simulink model "Hybrid_P2_Parallel_ETE"  (R2017b)
settings: Solver=FixedStepAuto  StartTime=0.0  StopTime=length(Speed)  FixedStep=0.01  MaxStep=0.01  RelTol=1e-3  EnableMultiTasking=on
PostLoadFcn:
  | , if any(exist('dsrtsu_mdlpostloadfcn', 'file') == [2, 3, 6]), try dsrtsu_mdlpostloadfcn('Execute', bdroot); catch fprintf('Error in PostLoadFcn (dsrtsu_mdlpostloadfcn) for model "%s":\n %s\n', bdroot, lasterr); end, end,
undefined symbols (not defined in the file): Actuators, APP1_OOR, APP2_OOR, APP_Mismatch, Brk_Flt, cal, ClutchEngag, CycLength, CycNmb, DiscIntNeverNeededParam, eng, Engine, EngOverTemp, ENGTRQ_MSMCH_Degraded_CP, ENGTRQ_MSMCH_ErrCritical_CP, ENGTRQ_MSMCH_LimpHome_CP, EngTrqMismatch, ess, ESSOverTemp, gb, Gearbox, KeyPos_Flt, lib_Actuators, lib_EMachine_2017a, lib_Sensors_2017a, Loss, LossCAN, Machine, MCUOverTemp, mot, MotDirMismatch, MotOverTemp, MotTrqMismatch, PRNDL_Flt, Ratio, RegenFault, Scope_new, Scopes1, Sensors, Spd, StopIndex, t_amb, time, tloop
libraries: simulink x117, EC2_libraries x9, powerlib_meascontrol x2, CalculationGallon x1, lib_Chassis x1, lib_DCDC x1, lib_Differential x1, lib_HVESS x1, lib_Engine x1, lib_OBC x1, lib_Transmission x1, Transmission_Validation x1
(part 3 of 10)

== system Hybrid_P2_Parallel_ETE/Camaro Plant Model/Scopes1/AxlTrq_to_EngTrq2/Ratio Filter ==
  Ratio : Inport
  Abs : Abs
  Compare To Zero : simulink/Logic and Bit Operations/Compare To Zero  relop===  OutDataTypeStr=boolean
  Constant : Constant  Value=cal.Time.TrnsOvrllEstTrqRatioSwitch
  Mature_Delay : EC2_libraries/Mature_Delay
      settings: SourceProductName=The database C:\Users\vrajm\AppData\Roaming\MathWorks\MATLAB\R2017b\slblocks_master.db is locked, or a table in the database is locked. (database is locked)
  Memory1 : Memory  InitialCondition=1
  Switch1 : Switch  Threshold=1
  Switch2 : Switch  Threshold=1
  Filtered_Ratio : Outport
  wires:
  Switch2/1 -> Memory1/1, Filtered_Ratio/1  "gear_ratio"
  Memory1/1 -> Switch1/3
  Mature_Delay/1 -> Switch1/2
  Constant/1 -> Mature_Delay/2
  Switch1/1 -> Switch2/1
  Abs/1 -> Switch2/3, Switch1/1
  Compare To Zero/1 -> Switch2/2, Mature_Delay/1
  Ratio/1 -> Abs/1, Compare To Zero/1

== system Hybrid_P2_Parallel_ETE/Camaro Plant Model/Scopes1/AxlTrq_to_MtrTrq2/Ratio Filter ==
  Ratio : Inport
  Abs : Abs
  Compare To Zero : simulink/Logic and Bit Operations/Compare To Zero  relop===  OutDataTypeStr=boolean
  Constant : Constant  Value=cal.Time.TrnsOvrllEstTrqRatioSwitch
  Mature_Delay : EC2_libraries/Mature_Delay
      settings: SourceProductName=The database C:\Users\vrajm\AppData\Roaming\MathWorks\MATLAB\R2017b\slblocks_master.db is locked, or a table in the database is locked. (database is locked)
  Memory1 : Memory  InitialCondition=1
  Switch1 : Switch  Threshold=1
  Switch2 : Switch  Threshold=1
  Filtered_Ratio : Outport
  wires:
  Switch2/1 -> Memory1/1, Filtered_Ratio/1  "gear_ratio"
  Memory1/1 -> Switch1/3
  Mature_Delay/1 -> Switch1/2
  Constant/1 -> Mature_Delay/2
  Switch1/1 -> Switch2/1
  Abs/1 -> Switch2/3, Switch1/1
  Compare To Zero/1 -> Switch2/2, Mature_Delay/1
  Ratio/1 -> Abs/1, Compare To Zero/1

== system Hybrid_P2_Parallel_ETE/Camaro Plant Model/Scopes1/Subsystem/StopCondition  ==
  note: Change the Cycle repeating to triggering repeatition,
      | and add the cycle repeated numbers
  BMS_SOC : Inport
  Gallon_fuel : Inport  Port=2
  10 gallons : simulink/Logic and Bit Operations/Compare To Constant  relop=>=  const=10  OutDataTypeStr=boolean
  Clock : Clock
  Compare To Constant2 : simulink/Logic and Bit Operations/Compare To Constant  relop===  const=4  OutDataTypeStr=boolean
  Constant : Constant  Value=CycNmb
  Constant1 : Constant  Value=0
  Constant2 : Constant  Value=StopIndex
  Constant3 : Constant  Value=CycLength
  Multiport Switch : MultiPortSwitch  Inputs=4
  Product : Product
  Relational Operator : RelationalOperator  Operator===  OutDataTypeStr=boolean  RndMeth=Simplest
  Stop Simulation : Stop
  "stop " : Subsystem
  wires:
  Constant3/1 -> Product/2
  Product/1 -> Relational Operator/2
  Constant1/1 -> Multiport Switch/5
  Relational Operator/1 -> Multiport Switch/4
  Constant/1 -> Product/1
  Gallon_fuel/1 -> 10 gallons/1
  Compare To Constant2/1 -> Multiport Switch/2
  "stop "/1(Out1) -> Compare To Constant2/1
  10 gallons/1 -> Multiport Switch/3
  BMS_SOC/1 -> "stop "/1(In1)
  Constant2/1 -> Multiport Switch/1
  Multiport Switch/1 -> Stop Simulation/1
  Clock/1 -> Relational Operator/1

== system Hybrid_P2_Parallel_ETE/Camaro Plant Model/Transmission/Inputs/Analog_fromHCU ==
  Outputs : Outport
  wires:
  [Analog] -> Outputs/1

== system Hybrid_P2_Parallel_ETE/Camaro Plant Model/Transmission/Inputs/CAN_fromHCU ==
  Outputs : Outport
  wires:
  [HCU_to_VEH_CAN] -> Outputs/1

== system Hybrid_P2_Parallel_ETE/Camaro Plant Model/Transmission/Inputs/Digital_fromHCU ==
  Outputs : Outport
  wires:
  [Digital] -> Outputs/1

== system Hybrid_P2_Parallel_ETE/Camaro Plant Model/Transmission/Soft TCM/6L45 Logic/Gearbox_Control.Shift_Schedule.PlotShiftSchedule ==
  f : TriggerPort  TriggerType=function-call  VariantControl=Variant
      settings: CopyFcn=Stateflow.SLINSF.SimulinkMan.removeBlockPreDeleteFcn  PreDeleteFcn=Stateflow.SLINSF.SimulinkMan.unsafePredeleteFcn
  Subsystem : Subsystem
      settings: OpenFcn=|
      | figure;
      | PlotGearShiftSchedule(Gearbox.L45.PedalPositions,Gearbox.L45.UpShiftSpeeds,Gearbox.L45.DownShiftSpeeds,'6L45')
      mask Display: disp('Plot')

== system Hybrid_P2_Parallel_ETE/Camaro Plant Model/Transmission/Soft TCM/6L45 Logic/Gearbox_Control.Shift_Schedule.calc_down ==
  Gear : Inport
  APP : Inport  Port=2
  f : TriggerPort  TriggerType=function-call  VariantControl=Variant
      settings: CopyFcn=Stateflow.SLINSF.SimulinkMan.removeBlockPreDeleteFcn  PreDeleteFcn=Stateflow.SLINSF.SimulinkMan.unsafePredeleteFcn
  Calculate Downshift Threshold : Lookup2D  RowIndex=gb.ctrl.dmd.init.gear_dnshift.idx1_lin_accel  ColumnIndex=[2,3,4,5,6,7,8]  Table=gb.ctrl.dmd.init.gear_dnshift.map'  LookUpMeth=Interpolation-Use End Values
  down_th : Outport
  wires:
  Calculate Downshift Threshold/1 -> down_th/1
  Gear/1 -> Calculate Downshift Threshold/2
  APP/1 -> Calculate Downshift Threshold/1

== system Hybrid_P2_Parallel_ETE/Camaro Plant Model/Transmission/Soft TCM/6L45 Logic/Gearbox_Control.Shift_Schedule.calc_up ==
  Gear : Inport
  APP : Inport  Port=2
  f : TriggerPort  TriggerType=function-call  VariantControl=Variant
      settings: CopyFcn=Stateflow.SLINSF.SimulinkMan.removeBlockPreDeleteFcn  PreDeleteFcn=Stateflow.SLINSF.SimulinkMan.unsafePredeleteFcn
  Calculate Upshift Threshold : Lookup2D  RowIndex=gb.ctrl.dmd.init.gear_upshift.idx1_lin_accel  ColumnIndex=[1,2,3,4,5,6,7]  Table=gb.ctrl.dmd.init.gear_upshift.map'  LookUpMeth=Interpolation-Use End Values
  up_th : Outport
  wires:
  Calculate Upshift Threshold/1 -> up_th/1
  APP/1 -> Calculate Upshift Threshold/1
  Gear/1 -> Calculate Upshift Threshold/2

== system Hybrid_P2_Parallel_ETE/Camaro Plant Model/Transmission/Soft TCM/6L45 Logic/Torque_Converter_Control.calc_lockup ==
  Gear : Inport
  APP : Inport  Port=2
  f : TriggerPort  TriggerType=function-call  VariantControl=Variant
      settings: CopyFcn=Stateflow.SLINSF.SimulinkMan.removeBlockPreDeleteFcn  PreDeleteFcn=Stateflow.SLINSF.SimulinkMan.unsafePredeleteFcn
  Calculate Lockup Threshold : Lookup2D  RowIndex=cpl.ctrl.init.trqconv_lockup.idx1_lin_accel  ColumnIndex=cpl.ctrl.init.trqconv_lockup.idx2_gear  Table=cpl.ctrl.init.trqconv_lockup.map  LookUpMeth=Interpolation-Use End Values
  lockup_th : Outport
  wires:
  Calculate Lockup Threshold/1 -> lockup_th/1
  APP/1 -> Calculate Lockup Threshold/1
  Gear/1 -> Calculate Lockup Threshold/2

== system Hybrid_P2_Parallel_ETE/Camaro Plant Model/Transmission/Soft TCM/6L45 Logic/Torque_Converter_Control.calc_unlock ==
  Gear : Inport
  APP : Inport  Port=2
  f : TriggerPort  TriggerType=function-call  VariantControl=Variant
      settings: CopyFcn=Stateflow.SLINSF.SimulinkMan.removeBlockPreDeleteFcn  PreDeleteFcn=Stateflow.SLINSF.SimulinkMan.unsafePredeleteFcn
  Calculate Unlock Threshold : Lookup2D  RowIndex=cpl.ctrl.init.trqconv_unlock.idx1_lin_accel  ColumnIndex=cpl.ctrl.init.trqconv_unlock.idx2_gear  Table=cpl.ctrl.init.trqconv_unlock.map  LookUpMeth=Interpolation-Use End Values
  unlock_th : Outport
  wires:
  Calculate Unlock Threshold/1 -> unlock_th/1
  APP/1 -> Calculate Unlock Threshold/1
  Gear/1 -> Calculate Unlock Threshold/2

== system Hybrid_P2_Parallel_ETE/Camaro Plant Model/Transmission/Transmission Plant/ Actuators ==
  In1 : Inport
  Bus Selector : BusSelector  OutputSignals=TransEstGear,LockupCmd
  Out2 : Outport
  Out5 : Outport  Port=2
  wires:
  In1/1 -> Bus Selector/1
  Bus Selector/1 -> Out2/1  "<TransEstGear>"
  Bus Selector/2 -> Out5/1  "<LockupCmd>"

== system Hybrid_P2_Parallel_ETE/Camaro Plant Model/Transmission/Transmission Plant/Gearbox ==
  TransEstGear : Inport
  gb_trq_in gb_inertia_in : Inport  Port=2
  gb_spd_out : Inport  Port=3
  Bus Creator : BusCreator  Inputs=2
  Bus Selector : BusSelector  OutputSignals=tc_trq_out,tc_inertia_out
  Engine Inertia : Constant  Value=Engine.Inertia
  Gear : Lookup  InputValues=gb.plant.init.gear.idx1_shifter  Table=gb.plant.init.gear.idx2_gear  LookUpMeth=Interpolation-Use End Values  OutDataTypeStr=double  SaturateOnIntegerOverflow=on
  Inertia Calculation : Subsystem
  Memory : Memory
  Speed Calculation : Subsystem
  Subsystem : Subsystem
  To Workspace : ToWorkspace  VariableName=TOSS  SampleTime=-1
  Torque calculation : Subsystem
  gear ratio table : Lookup  InputValues=gb.plant.init.ratio.idx1_gear  Table=gb.plant.init.ratio.map  LookUpMeth=Interpolation-Use End Values  SaturateOnIntegerOverflow=on
  "shaftspeed " : lib_Transmission/Transmission/Transmission Plant/Gearbox/shaftspeed 
  gb_trq_out gb_inertia_out : Outport
  gb_spd_in : Outport  Port=2
  tag scope: gb_gear=global, gb_inertia_in=global, gb_inertia_out=global, gb_spd_in=global, gb_spd_out=global, gb_trq_in=global, gb_trq_out=global, gb_trq_ratio=global
  wires:
  Bus Selector/2 -> Inertia Calculation/1(Inertia_in), Speed Calculation/4(Inertia Input)  "<tc_inertia_out>"
  Engine Inertia/1 -> [gb_inertia_in]
  Subsystem/1(Out1) -> [gb_trq_out], Bus Creator/1  "gb_trq_out"
  Torque calculation/1(torque_out) -> Subsystem/1(In1), Subsystem/2(In2)  "gb_trq_out"
  Memory/1 -> Gear/1
  gear ratio table/1 -> [gb_trq_ratio]
  Bus Creator/1 -> gb_trq_out gb_inertia_out/1
  Inertia Calculation/1(Inertia) -> Bus Creator/2, [gb_inertia_out]  "gb_inertia_out"
  gb_trq_in gb_inertia_in/1 -> Bus Selector/1
  Gear/1 -> Torque calculation/2(gear number), Inertia Calculation/2(gear number), gear ratio table/1, [gb_gear], Speed Calculation/1(gear number)
  Bus Selector/1 -> Torque calculation/3(" input torque"), Speed Calculation/3(torque input), [gb_trq_in]  "<tc_trq_out>"
  TransEstGear/1 -> Memory/1
  Speed Calculation/1(Speed) -> gb_spd_in/1, "shaftspeed "/1, [gb_spd_in]
  gb_spd_out/1 -> Speed Calculation/2(spd out), "shaftspeed "/2, [gb_spd_out], To Workspace/1, Torque calculation/1(speed out)

== system Hybrid_P2_Parallel_ETE/Camaro Plant Model/Transmission/Transmission Plant/Sensors ==
  In2 : Inport
  In3 : Inport  Port=2
  In4 : Inport  Port=3
  In5 : Inport  Port=4
  In6 : Inport  Port=5
  In7 : Inport  Port=6
  In1 : Inport  Port=7
  Bus Creator : BusCreator  Inputs=7
  Out1 : Outport
  wires:
  In1/1 -> Bus Creator/7  "gb_trq_ratio"
  Bus Creator/1 -> Out1/1
  In2/1 -> Bus Creator/1  "impeller_spd_rads"
  In4/1 -> Bus Creator/3  "tc_trq_in"
  In5/1 -> Bus Creator/4  "tc_trq_out"
  In3/1 -> Bus Creator/2  "turbine_spd_rads"
  In6/1 -> Bus Creator/5  "TrnsOutShftAngVel"
  In7/1 -> Bus Creator/6  "TrnsOutShftTrq"

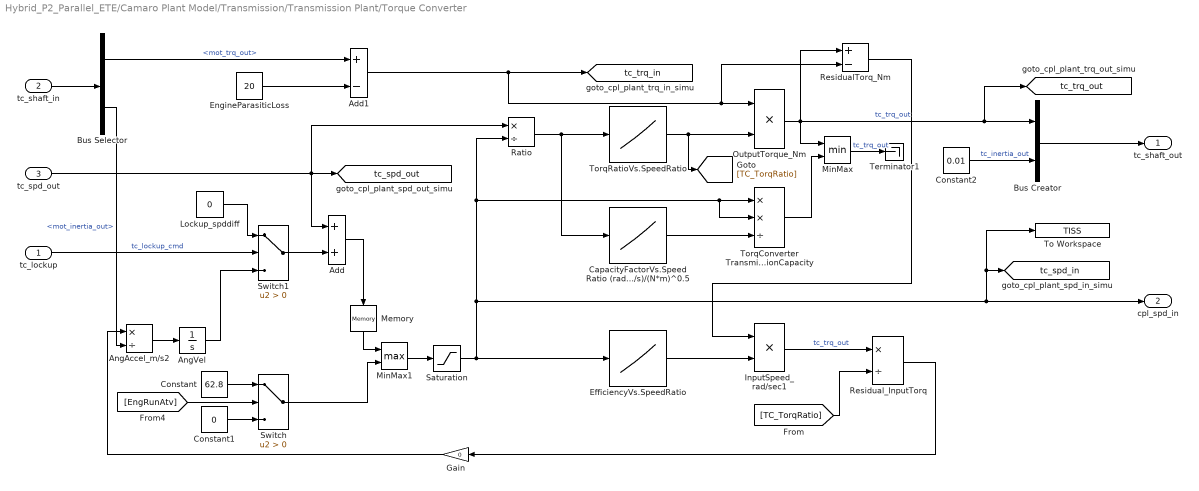
== system Hybrid_P2_Parallel_ETE/Camaro Plant Model/Transmission/Transmission Plant/Torque Converter ==
  tc_lockup : Inport
  tc_shaft_in : Inport  Port=2
  tc_spd_out : Inport  Port=3
  Add : Sum
  Add1 : Sum  Inputs=+-
  AngAccel_m/s2 : Product  Inputs=*/
  AngVel : Integrator
  Bus Creator : BusCreator  Inputs=2
  Bus Selector : BusSelector  OutputSignals=mot_trq_out,mot_inertia_out
  CapacityFactorVs.SpeedRatio (rad/s)/(N*m)^0.5 : Lookup_n-D  NumberOfTableDimensions=1  BreakpointsForDimension1=[0 0.50 0.60 0.70 0.80 0.87 0.92 0.94 0.96 0.97]  Table=[12.2938 12.8588 13.1452 13.6285 14.6163 16.2675 19.3503 22.1046 29.9986 50.00]  InternalRulePriority=Speed  RndMeth=Simplest  InputSameDT=on
  Constant : Constant  Value=62.8
  Constant1 : Constant  Value=0
  Constant2 : Constant  Value=0.01
  EfficiencyVs.SpeedRatio : Lookup_n-D  NumberOfTableDimensions=1  BreakpointsForDimension1=[0 0.25 0.50 0.60 0.70 0.80 0.87 0.92 0.94 0.96 0.97 1.0]  Table="[0.10 0.50 0.70 0.8 0.8 0.80  0.85 0.87 0.91 0.95 0.96 0.96]"  InternalRulePriority=Speed  RndMeth=Simplest  InputSameDT=on
  EngineParasiticLoss : Constant  Value=20
  Gain : Gain  Gain=0
  InputSpeed_rad/sec1 : Product  Inputs=**
  Lockup_spddiff : Constant  Value=0
  Memory : Memory  InitialCondition=1
  MinMax : MinMax  Inputs=2
  MinMax1 : MinMax  Function=max  Inputs=2
  OutputTorque_Nm : Product  Inputs=**
  Ratio : Product  Inputs=*/
  ResidualTorq_Nm : Sum  Inputs=+-
  Residual_InputTorq : Product  Inputs=*/
  Saturation : Saturate  UpperLimit=1100  LowerLimit=1
  Switch : Switch  Criteria=u2 > Threshold
  Switch1 : Switch  Criteria=u2 > Threshold
  Terminator1 : Terminator
  To Workspace : ToWorkspace  VariableName=TISS  SampleTime=-1
  TorqConverter TransmissionCapacity : Product  Inputs=**/
  TorqRatioVs.SpeedRatio : Lookup_n-D  NumberOfTableDimensions=1  BreakpointsForDimension1=[0 0.50 0.60 0.70 0.80 0.87 0.92 0.94 0.96 0.97]  Table=[2.2320 1.5462 1.4058 1.2746 1.1528 1.0732 1.0192 0.9983 0.9983 0.9983]  InternalRulePriority=Speed  RndMeth=Simplest  InputSameDT=on
  tc_shaft_out : Outport
  cpl_spd_in : Outport  Port=2
  tag scope: tc_spd_in=global, tc_spd_out=global, tc_trq_in=global, tc_trq_out=global
  wires:
  Lockup_spddiff/1 -> Switch1/1
  Switch1/1 -> Add/2
  Bus Selector/1 -> Add1/1  "<mot_trq_out>"
  Constant1/1 -> Switch/3
  Constant/1 -> Switch/1
  [EngRunAtv] -> Switch/2
  Switch/1 -> MinMax1/2
  MinMax1/1 -> Saturation/1
  Gain/1 -> AngAccel_m/s2/1
  Add/1 -> Memory/1
  tc_spd_out/1 -> Add/1, [tc_spd_out], Ratio/1
  MinMax/1 -> Terminator1/1  "tc_trq_out"
  OutputTorque_Nm/1 -> MinMax/1, [tc_trq_out], Bus Creator/1, ResidualTorq_Nm/1  "tc_trq_out"
  Residual_InputTorq/1 -> Gain/1
  EngineParasiticLoss/1 -> Add1/2
  Memory/1 -> MinMax1/1
  AngVel/1 -> Switch1/3
  AngAccel_m/s2/1 -> AngVel/1
  InputSpeed_rad/sec1/1 -> Residual_InputTorq/1  "tc_trq_out"
  ResidualTorq_Nm/1 -> InputSpeed_rad/sec1/1
  [TC_TorqRatio] -> Residual_InputTorq/2
  TorqConverter TransmissionCapacity/1 -> MinMax/2
  EfficiencyVs.SpeedRatio/1 -> InputSpeed_rad/sec1/2
  Saturation/1 -> EfficiencyVs.SpeedRatio/1, cpl_spd_in/1, To Workspace/1, [tc_spd_in], TorqConverter TransmissionCapacity/1, TorqConverter TransmissionCapacity/2, Ratio/2
  Ratio/1 -> TorqRatioVs.SpeedRatio/1, CapacityFactorVs.SpeedRatio (rad/s)/(N*m)^0.5/1
  CapacityFactorVs.SpeedRatio (rad/s)/(N*m)^0.5/1 -> TorqConverter TransmissionCapacity/3
  TorqRatioVs.SpeedRatio/1 -> [TC_TorqRatio], OutputTorque_Nm/2
  tc_lockup/1 -> Switch1/2  "tc_lockup_cmd"
  Bus Selector/2 -> AngAccel_m/s2/2  "<mot_inertia_out>"
  Bus Creator/1 -> tc_shaft_out/1
  tc_shaft_in/1 -> Bus Selector/1
  Constant2/1 -> Bus Creator/2  "tc_inertia_out"
  Add1/1 -> OutputTorque_Nm/1, ResidualTorq_Nm/2, [tc_trq_in]

== system Hybrid_P2_Parallel_ETE/Controller_with_Transmission_Manager1/HSC/Camaro Fault Detection/Component Diagnostic ==
  note: Component Diagnostics
  note: Component Status Setting Rule
      | xxx_CompStatus could be 0, 1, 2 or 3
      | 0: component needs to be offline
      | 1: component needs torque plant to deliver creep torque
      | 2: component needs torque plant to limit maximum torque delivery
      | 3: component needs torque plant to operate normally
  SignalDiag : Inport
  Bus Creator : BusCreator  Inputs=6
  Driver Input Diagnostic : Subsystem
  ESS Component Diagnostic : Subsystem
  Engine Component Diagnostic : Subsystem
  Override Driver Status : Subsystem
  Override ESS Status : Subsystem
  Override Engine Status : Subsystem
  Override TCM Status : Subsystem
  Transmission Component Diagnostic : Subsystem
  CompDiag : Outport
  wires:
  Engine Component Diagnostic/2(Out2) -> Bus Creator/4  "EngTrqMismchType"
  Override Driver Status/1(Out1) -> Bus Creator/1  "Driver_Input_Status"
  Override TCM Status/1(Out1) -> Bus Creator/5  "TCM_Status"
  Override Engine Status/1(Out1) -> Bus Creator/3  "ECM_Status"
  Override ESS Status/1(Out1) -> Bus Creator/2  "BMS_Status"
  Transmission Component Diagnostic/1(Out1) -> Override TCM Status/1(In1)  "TCM_CompDiag"
  Engine Component Diagnostic/1(Out1) -> Override Engine Status/1(In1)  "ECM_CompDiag"
  ESS Component Diagnostic/1(Out1) -> Override ESS Status/1(In1)  "ESS_CompDiag"
  Driver Input Diagnostic/1(Out1) -> Override Driver Status/1(In1)  "Diver_CompDiag"
  Bus Creator/1 -> CompDiag/1
  SignalDiag/1 -> Driver Input Diagnostic/1(In1), ESS Component Diagnostic/1(In1), Bus Creator/6, Transmission Component Diagnostic/1(In1), Engine Component Diagnostic/1(In1)  "RawSig"

== system Hybrid_P2_Parallel_ETE/Controller_with_Transmission_Manager1/HSC/Camaro Fault Detection/Input Conversions ==
  note: These subsystems convert variable types to match those used in the
      | supervisor. In addition, override switches installed on each signal can
      | be used to manually override and signal for testing purposes
  note: Input Conversions and Override Switches
  RawSig : Inport
  BMS_Conversions : Subsystem
  Bus Creator : BusCreator  Inputs=5
  DriverInput_Conversions : Subsystem
  ECM_Conversions : Subsystem
  TCM_Conversions : Subsystem
  VehSig : Outport
  wires:
  TCM_Conversions/1(Out1) -> Bus Creator/4
  ECM_Conversions/1(Out1) -> Bus Creator/3
  RawSig/1 -> BMS_Conversions/1(In1), ECM_Conversions/1(In1), TCM_Conversions/1(In1), Bus Creator/5, DriverInput_Conversions/1(In1)  "RawSig"
  BMS_Conversions/1(Out1) -> Bus Creator/2
  Bus Creator/1 -> VehSig/1  "InputConvAndOvrd"
  DriverInput_Conversions/1(Out1) -> Bus Creator/1

== system Hybrid_P2_Parallel_ETE/Controller_with_Transmission_Manager1/HSC/Camaro Fault Detection/Signal Diagnostic ==
  note: Signal Diagnostics
  note: These subsystems evaluate each signal for proper value range and other checks
  VehSig : Inport
  Bus Creator : BusCreator  Inputs=5
  Driver Signal Diagnostic : Subsystem
  ESS Signal Diagnostic : Subsystem
  Engine Signal Diagnostic : Subsystem
  Subsystem1 : Subsystem
      mask Display: fprintf('Signal Naming Rule')
  Transmission Signal Diagnostic : Subsystem
  SignalDiag : Outport
  wires:
  Bus Creator/1 -> SignalDiag/1  "SignalDiag"
  Transmission Signal Diagnostic/1(Out2) -> Bus Creator/4  "Transmission_SigDiag"
  Engine Signal Diagnostic/1(Engine_SigDiag) -> Bus Creator/3  "Engine_SigDiag"
  ESS Signal Diagnostic/1(ESS_SigDiag) -> Bus Creator/2  "ESS_SigDiag"
  Driver Signal Diagnostic/1(Driver_SigDiag) -> Bus Creator/1  "Driver_SigDiag"
  VehSig/1 -> Transmission Signal Diagnostic/1(Sensors1), Bus Creator/5, Engine Signal Diagnostic/1(Sensors1), Driver Signal Diagnostic/1(Sensors1), ESS Signal Diagnostic/1(Sensors1)

== system Hybrid_P2_Parallel_ETE/Controller_with_Transmission_Manager1/HSC/Driver_Requests/APP_BPP to DrvIntndAxlTrq2 ==
  note: Note:Driver requested Axle Torque Calculation
  note: $Author: fy6949 $
      | $Rev: 577 $
      | $Date: 2017-1-19 08:53:15 -0500  $
  Sensors : Inport
  Diag : Inport  Port=2
  Controls : Inport  Port=3
  Bus Selector : BusSelector  OutputSignals=from_Analog.Driver_APP1,from_CAN.fromVEH_CAN.from_BCM.BrkPdlPos,from_CAN.fromEBCAN.from_ECM.VehSpdAvgDrvn,from_CAN.fromVEH_CAN.from_TCM.TrnGrRat,from_CAN.fromHV_CAN.from_MCU.INV_VCU_01.INV_Speed
  Bus Selector1 : BusSelector  OutputSignals=CompSig.RawSig.Driver_SigDiag.Drv_APP_Agree
  Bus Selector2 : BusSelector  OutputSignals=mode
  Post Driver Intnded Axle Torque : Subsystem
  Terminator : Terminator
  Terminator1 : Terminator
  IntndAxlTrq : Outport
  wires:
  Sensors/1 -> Bus Selector/1
  Controls/1 -> Bus Selector2/1
  Post Driver Intnded Axle Torque/1(IntndAxlTrq) -> IntndAxlTrq/1
  Bus Selector/2 -> Post Driver Intnded Axle Torque/2(BPP)  "<BrkPdlPos>"
  Bus Selector/3 -> Post Driver Intnded Axle Torque/3(VehicleSpeed)  "<VehSpdAvgDrvn>"
  Bus Selector/5 -> Post Driver Intnded Axle Torque/6(Motor_Speed)  "<INV_Speed>"
  Bus Selector/4 -> Post Driver Intnded Axle Torque/4(TransGearRatio)  "<TrnGrRat>"
  Bus Selector/1 -> Post Driver Intnded Axle Torque/1(APP)  "<Driver_APP1>"
  Post Driver Intnded Axle Torque/2(BrkIntndAxlTrq) -> Terminator/1
  Diag/1 -> Bus Selector1/1
  Bus Selector1/1 -> Terminator1/1  "<Drv_APP_Agree>"
  Bus Selector2/1 -> Post Driver Intnded Axle Torque/5(Mode)  "<mode>"

== system Hybrid_P2_Parallel_ETE/Controller_with_Transmission_Manager1/HSC/Powertrain Manager/HV Manager1 ==
  Sensors : Inport
  Controls : Inport  Port=2
  Axiomatic_Output_Manager : Subsystem
  BMS_Manager : Subsystem
  Bus Creator1 : BusCreator  Inputs=4
  DCDC Manager : Subsystem
  Inverter Manager : Subsystem
  OBC_Manager : Subsystem
  BMS_CAN : Outport
  HV_BUS_Status : Outport  Port=2
  OBC_CAN : Outport  Port=3
  OBC_Digital : Outport  Port=4
  BMS_Digital : Outport  Port=5
  Axiomatic_CAN : Outport  Port=6
  tag scope: MCU_CAN=global
  wires:
  Bus Creator1/1 -> [MCU_CAN]
  Inverter Manager/2(MCU_CAN) -> Bus Creator1/2  "MCU_CAN"
  Inverter Manager/1(MCU_Status) -> [MCU_Status], Bus Creator1/1  "MCU_Status"
  Sensors/1 -> BMS_Manager/1(Sensors), DCDC Manager/1(BMSInput), Axiomatic_Output_Manager/1(Sensors), OBC_Manager/2(Sensors), Inverter Manager/2(Sensors)
  [HV_BUS_Status] -> Inverter Manager/1(HV_Bus_Status)  "HV_BUS_Status"
  [HV_BUS_Status] -> Axiomatic_Output_Manager/2(HV_Bus_Status)
  BMS_Manager/2(HV_BUS_Status) -> [HV_BUS_Status], HV_BUS_Status/1  "HV_BUS_Status"
  [HV_BUS_Status] -> OBC_Manager/1(HV_Status)
  OBC_Manager/1(OBC CAN) -> OBC_CAN/1
  OBC_Manager/2(OBC_Digital) -> OBC_Digital/1
  Controls/1 -> BMS_Manager/2(Controls), DCDC Manager/2(In1), DCDC Manager/3(In2), Inverter Manager/3(Control)
  BMS_Manager/1(BMS CAN) -> BMS_CAN/1
  BMS_Manager/3(BMS Digital) -> BMS_Digital/1
  Axiomatic_Output_Manager/1(Axiomatic_CAN) -> Axiomatic_CAN/1
  Inverter Manager/3(MCU_Relay) -> Bus Creator1/3  "MCU_Relay"
  DCDC Manager/1(Out1) -> Bus Creator1/4
  [MCU_Status] -> BMS_Manager/3(In1)

== system Hybrid_P2_Parallel_ETE/Controller_with_Transmission_Manager1/HSC/Powertrain Manager/Output Conversion ==
  In1 : Inport
  In2 : Inport  Port=2
  In3 : Inport  Port=3
  In4 : Inport  Port=4
  In5 : Inport  Port=5
  In8 : Inport  Port=6
  In9 : Inport  Port=7
  In10 : Inport  Port=8
  In11 : Inport  Port=9
  Bus Creator : BusCreator  Inputs=14
  Bus Creator1 : BusCreator  Inputs=9
  Bus Selector2 : BusSelector  OutputSignals=powerMode,EnablePrplsn,ClutchEngage,EngAppReq,EngOnReq,MtrTrqCmdOut,EnableInverter,EngTrqCmd,HV_req,SysPwrMd_0_3,TrnsShftLvrPos,VehSpdAvgDrvn_kph,AccPos_Perc,SportsModeEnable
  Data Type Conversion{,2..3,5..13} (12 alike) : DataTypeConversion
  Memory : Memory
  Out1 : Outport
  wires:
  In10/1 -> Bus Creator1/8
  In9/1 -> Bus Creator1/7
  In8/1 -> Bus Creator1/6
  Memory/1 -> Data Type Conversion/1
  Data Type Conversion13/1 -> Bus Creator/13  "AccPos_Perc"
  Bus Selector2/13 -> Data Type Conversion13/1  "<AccPos_Perc>"
  Data Type Conversion12/1 -> Bus Creator/12  "VehSpdAvgDrvn_kph"
  Bus Selector2/12 -> Data Type Conversion12/1  "<VehSpdAvgDrvn_kph>"
  Data Type Conversion11/1 -> Bus Creator/11  "ShftLvrPos"
  Bus Selector2/11 -> Data Type Conversion11/1  "<TrnsShftLvrPos>"
  In5/1 -> Bus Creator1/5
  Bus Creator/1 -> Bus Creator1/4  "Controls"
  In3/1 -> Bus Creator1/3
  In2/1 -> Bus Creator1/2
  In1/1 -> Bus Creator1/1
  Bus Creator1/1 -> Out1/1
  Data Type Conversion5/1 -> Bus Creator/5  "EngOnReq"
  Data Type Conversion/1 -> Bus Creator/1  "powerMode"
  Data Type Conversion10/1 -> Bus Creator/10  "SysPwrMd"
  Data Type Conversion9/1 -> Bus Creator/9  "HV_req"
  Data Type Conversion8/1 -> Bus Creator/8  "EngTrqCmd"
  Data Type Conversion7/1 -> Bus Creator/7  "Inverter_Enable"
  Data Type Conversion6/1 -> Bus Creator/6  "Torque_Command"
  Bus Selector2/4 -> Bus Creator/4  "<EngAppReq>"
  Data Type Conversion3/1 -> Bus Creator/3  "ClutchEngage"
  Data Type Conversion2/1 -> Bus Creator/2  "EnablePrplsn"
  Bus Selector2/10 -> Data Type Conversion10/1  "<SysPwrMd_0_3>"
  Bus Selector2/9 -> Data Type Conversion9/1  "<HV_req>"
  Bus Selector2/8 -> Data Type Conversion8/1  "<EngTrqCmd>"
  Bus Selector2/7 -> Data Type Conversion7/1  "<EnableInverter>"
  Bus Selector2/6 -> Data Type Conversion6/1  "<MtrTrqCmdOut>"
  Bus Selector2/5 -> Data Type Conversion5/1  "<EngOnReq>"
  Bus Selector2/3 -> Data Type Conversion3/1  "<ClutchEngage>"
  Bus Selector2/2 -> Data Type Conversion2/1  "<EnablePrplsn>"
  Bus Selector2/1 -> Memory/1  "<powerMode>"
  In4/1 -> Bus Selector2/1
  In11/1 -> Bus Creator1/9
  Bus Selector2/14 -> Bus Creator/14  "<SportsModeEnable>"

== system Hybrid_P2_Parallel_ETE/Controller_with_Transmission_Manager1/HSC/Powertrain Manager/Thermal Manager ==
  In2 : Inport
  Bus Creator : BusCreator  Inputs=3
  Bus Creator1 : BusCreator  Inputs=4
  Bus Creator2 : BusCreator  Inputs=4
  Bus Creator3 : BusCreator  Inputs=3
  Bus Creator4 : BusCreator  Inputs=1
  Bus Selector : BusSelector  OutputSignals=from_CAN.fromEBCAN.from_ECM.EngCltTmp,from_CAN.fromHV_CAN.from_BMSHybrid.BMS_Temperatur,from_CAN.fromHV_CAN.from_MCU.INV_VCU_04.INV_InverterTemperature,from_CAN.fromHV_CAN.from_MCU.INV_VCU_04.INV_ElectricMachineTemperature,from_CAN.fromEBCAN.from_ECM.EngRunAtv,from_CAN.fromHV_CAN.from_BMSHybrid.BMS_HYB_02.BMS_IstModus,from_CAN.fromVEH_CAN.from_BCM.SysPwrMd,from_CAN.fromEBCAN.from_ECM.VehSpdAvgDrvn
  Bus Selector3 : BusSelector  OutputSignals=from_CAN.fromHV_CAN.from_BMSHybrid.BMS_HYB_02.BMS_Fehler_Pilot
  Compare To Constant1 : simulink/Logic and Bit Operations/Compare To Constant  relop=>  const=0  OutDataTypeStr=boolean
  Cooling Fan Manger : Subsystem
  Data Type Conversion : DataTypeConversion  OutDataTypeStr=double
  ESS Pump Manger : Subsystem
  MotInv Pump Manger : Subsystem
  Out1 : Outport
  wires:
  Bus Selector/8 -> Bus Creator/3  "<VehSpdAvgDrvn>"
  Bus Selector/7 -> Bus Creator3/3  "<SysPwrMd>"
  Bus Selector/6 -> Bus Creator3/2  "<BMS_IstModus>"
  Bus Selector/5 -> Bus Creator3/1  "<EngRunAtv>"
  Bus Selector/4 -> Bus Creator2/4  "<INV_ElectricMachineTemperature>"
  Bus Selector/3 -> Bus Creator2/3  "<INV_InverterTemperature>"
  Bus Selector/2 -> Bus Creator2/2  "<BMS_Temperatur>"
  Bus Selector/1 -> Bus Creator2/1  "<EngCltTmp>"
  Bus Creator1/1 -> Out1/1  "Thermal_Control"
  Cooling Fan Manger/1(Fan_control) -> Bus Creator1/1  "Fan_Control"
  Bus Creator/1 -> Cooling Fan Manger/1(Temp), ESS Pump Manger/1(ESS_temp), MotInv Pump Manger/1(MotInv_temp)
  ESS Pump Manger/1(ESS_Thermal_Control) -> Bus Creator1/2  "ESS_Pump_Control"
  MotInv Pump Manger/1(MotInvpump_control) -> Bus Creator1/3  "MotMCU_Pump_Control"
  Bus Creator2/1 -> Bus Creator/1  "Temp_Signals"
  Bus Creator3/1 -> Bus Creator/2  "Component_State"
  In2/1 -> Bus Selector3/1, Bus Selector/1
  Bus Selector3/1 -> Compare To Constant1/1  "<BMS_Fehler_Pilot>"
  Bus Creator4/1 -> Bus Creator1/4  "Pump_Commands"
  Data Type Conversion/1 -> Bus Creator4/1  "FuelPump_Disable"
  Compare To Constant1/1 -> Data Type Conversion/1

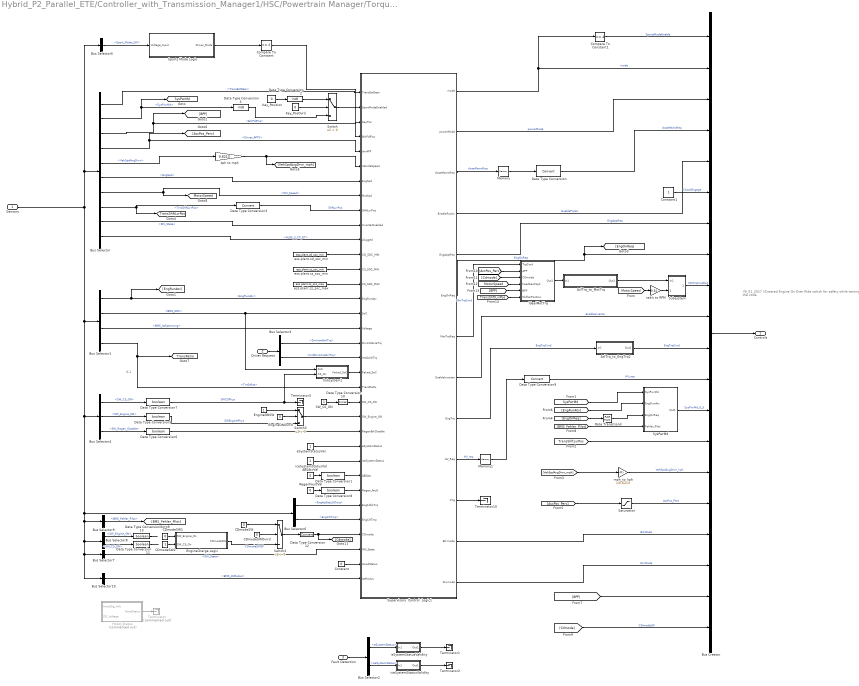
== system Hybrid_P2_Parallel_ETE/Controller_with_Transmission_Manager1/HSC/Powertrain Manager/Torque Distribution1 ==
  note: 0-1
  note: //9_01_2017
      | //Created Engine On Over Ride switch for safety while testing the code
  Sensors : Inport
  Driver Request : Inport  Port=2
  Fault Detection : Inport  Port=3
  ABSAtvVal : Constant  Value=0
  AxlTrq_to_EngTrq2 : Subsystem
  AxlTrq_to_MotTrq : Subsystem
  Bus Creator : BusCreator  Inputs=20
  Bus Selector : BusSelector  OutputSignals=from_CAN.fromVEH_CAN.from_TCM.TransEstGear,from_CAN.fromVEH_CAN.from_BCM.SysPwrMd,from_CAN.fromVEH_CAN.from_BCM.BrkPdlPos,from_Analog.Driver_APP1,from_CAN.fromEBCAN.from_ECM.VehSpdAvgDrvn,from_CAN.fromEBCAN.from_ECM.EngSpd,from_CAN.fromHV_CAN.from_MCU.INV_VCU_01.INV_Speed,from_CAN.fromVEH_CAN.from_TCM.TrnsShftLvrPos,from_CAN.fromHV_CAN.from_MCU.INV_VCU_01.INV_State,from_CAN.fromHV_CAN.from_OBC.NLG5_ST.NLG5_S_CP_DT
  Bus Selector1 : BusSelector  OutputSignals=from_CAN.fromEBCAN.from_ECM.EngRunAtv,from_CAN.fromHV_CAN.from_BMSHybrid.BMS_SOC,from_CAN.fromHV_CAN.from_BMSHybrid.BMS_HYB_02.BMS_IstSpannung,from_CAN.fromVEH_CAN.from_TCM.TrnGrRat
  Bus Selector10 : BusSelector  OutputSignals=from_CAN.fromHV_CAN.from_BMSHybrid.BMS_HYB_02.BMS_IstModus
  Bus Selector2 : BusSelector  OutputSignals=eSystemDiagOut.eSystemStatus,iceSystemDiagOut.iceSystemStatus
  Bus Selector3 : BusSelector  OutputSignals=DrvIntndAxlTrq,FullDrvIntndAxlTrq
  Bus Selector4 : BusSelector  OutputSignals=from_Digital.SW_CS_ON,from_Digital.SW_Engine_ON,from_Digital.SW_Regen_Disable
  Bus Selector5 : BusSelector  OutputSignals=from_Analog.Sport_Mode_SW
  Bus Selector6 : BusSelector  OutputSignals=from_CAN.fromEBCAN.from_ECM.EngActStdyStTorq,from_CAN.fromEBCAN.from_ECM.EngCltTmp
  Bus Selector7 : BusSelector  OutputSignals=from_CAN.fromHV_CAN.from_MCU.INV_VCU_01.INV_State
  Bus Selector8 : BusSelector  OutputSignals=from_Digital.SW_Engine_ON,from_Digital.SW_CS_ON
  Bus Selector9 : BusSelector  OutputSignals=from_CAN.fromHV_CAN.from_BMSHybrid.BMS_HYB_02.BMS_Fehler_Pilot
  CDmodeSW : Constant  Value=0
  CDmodeSW1 : Constant  Value=0
  CDmodeSW2 : Constant
  CDmodeSWOvrrd : Constant  Value=0
  Compare To Constant : simulink/Logic and Bit Operations/Compare To Constant  relop===  const=2  OutDataTypeStr=boolean
  Compare To Constant1 : simulink/Logic and Bit Operations/Compare To Constant  relop===  const=4  OutDataTypeStr=boolean
  Constant : Constant  Value=0
  Constant1 : Constant
  Data Type Conversion{,3,9,12} (4 alike) : DataTypeConversion
  Data Type Conversion{1,5..8,10..11,13} (8 alike) : DataTypeConversion  OutDataTypeStr=boolean
  Data Type Conversion2 : DataTypeConversion  OutDataTypeStr=int8
  Data Type Conversion4 : DataTypeConversion  OutDataTypeStr=int8
  EngineCharge Logic : Stateflow chart  TreatAsAtomicUnit=on
  EngineONOvrrd : Constant  Value=0
  EngineONSW : Constant
  Hood_Status : Subsystem  Commented=on
  IdealMotTrq : Subsystem
  Key_PosOvrd : Constant  Value=0
  Key_Position : Constant  Value=0
  Memory : Memory
  Memory1 : Memory
  Rate Transition3 : RateTransition
  RegenFaultVal : Constant  Value=0
  SW_CS_ON : Constant
  Saturation : Saturate  UpperLimit=100  LowerLimit=0
  Sports Mode Logic : Stateflow chart  TreatAsAtomicUnit=on
  Subsystem : Subsystem
  Subsystem1 : Subsystem
  Supervisory  Control  Logic1 : Stateflow chart  TreatAsAtomicUnit=on
  Switch : Switch  Criteria=u2 > Threshold
  Switch2 : Switch  Criteria=u2 > Threshold
  Switch3 : Switch  Criteria=u2 > Threshold
  SysPwrMd : Subsystem
  Terminator : Terminator  Commented=on
  Terminator{1..3,10} (4 alike) : Terminator
  eSystemStatusVal : Constant
  eSystemStatusValidity : Subsystem
  ess.plant.cd_soc_min : Constant  Value=ess.plant.cd_soc_min
  ess.plant.cs_soc_max : Constant  Value=ess.plant.cs_soc_max
  ess.plant.cs_soc_min : Constant  Value=ess.plant.cs_soc_min
  iceSystemStatusVal : Constant
  iceSystemStatusValidity : Subsystem
  kph to mph : Gain  Gain=0.6213
  mph_to_kph : Gain  Gain=1/0.6213
  rad/s to RPM : Gain  Gain=9.54
  Controls : Outport
  tag scope: MotorSpeed=global, SysPwrMd=global, TransRatio=global, TransShftLvrPos=global
  wires:
  Bus Selector/1 -> Supervisory  Control  Logic1/1(TransEstGear)  "<TransEstGear>"
  Bus Selector/2 -> [SysPwrMd], Data Type Conversion4/1  "<SysPwrMd>"
  Bus Selector/3 -> [BPP], Supervisory  Control  Logic1/4(BrkPdlPos)  "<BrkPdlPos>"
  Bus Selector/4 -> [AccPos_Perc], Supervisory  Control  Logic1/5(drvAPP)  "<Driver_APP1>"
  Bus Selector/5 -> kph to mph/1  "<VehSpdAvgDrvn>"
  Bus Selector/6 -> Supervisory  Control  Logic1/7(EngSpd)  "<EngSpd>"
  Bus Selector/7 -> [MotorSpeed], Supervisory  Control  Logic1/8(MotSpd)  "<INV_Speed>"
  Bus Selector/9 -> Supervisory  Control  Logic1/10(InverterEnabled)  "<INV_State>"
  Bus Selector1/1 -> Supervisory  Control  Logic1/15(EngRunAtv), [EngRunAtv]  "<EngRunAtv>"
  Bus Selector1/2 -> Subsystem1/1(SoC), Supervisory  Control  Logic1/16(SoC)  "<BMS_SOC>"
  ess.plant.cd_soc_min/1 -> Supervisory  Control  Logic1/12(CD_SOC_MIN)
  ess.plant.cs_soc_min/1 -> Supervisory  Control  Logic1/13(CS_SOC_MIN)
  ess.plant.cs_soc_max/1 -> Supervisory  Control  Logic1/14(CS_SOC_MAX)
  Supervisory  Control  Logic1/6(EngOnReq) -> [EngOnReq], Bus Creator/8  "EngOnReq"
  Supervisory  Control  Logic1/8(EnableInverter) -> Bus Creator/10  "EnableInverter"
  Supervisory  Control  Logic1/4(EnablePrplsn) -> Bus Creator/5  "EnablePrplsn"
  Supervisory  Control  Logic1/3(closeMaincReq) -> Memory/1  "closeMaincReq"
  Supervisory  Control  Logic1/2(powerMode) -> Bus Creator/3  "powerMode"
  Supervisory  Control  Logic1/1(mode) -> Compare To Constant1/1, Bus Creator/2  "mode"
  [EngOnReq] -> Rate Transition3/1
  [EngRunAtv] -> SysPwrMd/2(EngRunAtv)
  [SysPwrMd] -> SysPwrMd/1(SysPwrMd)
  Compare To Constant/1 -> Supervisory  Control  Logic1/2(SportModeEnabled)
  Data Type Conversion3/1 -> Supervisory  Control  Logic1/9(ShftLvrPos)  "ShftLvrPos"
  Bus Selector/8 -> [TransShftLvrPos], Data Type Conversion3/1  "<TrnsShftLvrPos>"
  kph to mph/1 -> [VehSpdAvgDrvn_mph], Supervisory  Control  Logic1/6(VehicleSpeed)
  Bus Creator/1 -> Controls/1
  Supervisory  Control  Logic1/9(EngTrq) -> AxlTrq_to_EngTrq2/1(In1)  "EngTrqCmd"
  Bus Selector1/4 -> Supervisory  Control  Logic1/21(TransRatio), [TransRatio]  "<TrnGrRat>"
  SysPwrMd/1(Out1) -> Bus Creator/13  "SysPwrMd_0_3"
  Supervisory  Control  Logic1/10(HV_Req) -> Memory1/1  "HV_req"
  [TransShftLvrPos] -> Bus Creator/14
  [VehSpdAvgDrvn_mph] -> mph_to_kph/1
  mph_to_kph/1 -> Bus Creator/15  "VehSpdAvgDrvn_kph"
  [AccPos_Perc] -> Saturation/1
  Saturation/1 -> Bus Creator/16  "AccPos_Perc"
  Driver Request/1 -> Bus Selector3/1
  Rate Transition3/1 -> SysPwrMd/3(EngOnReq)
  Constant1/1 -> Bus Creator/6  "ClutchEngage"
  AxlTrq_to_EngTrq2/1(Out1) -> Bus Creator/11  "EngTrqCmd"
  Fault Detection/1 -> Bus Selector2/1
  Bus Selector2/1 -> eSystemStatusValidity/1(In1)  "<eSystemStatus>"
  Bus Selector2/2 -> iceSystemStatusValidity/1(In1)  "<iceSystemStatus>"
  Bus Selector4/3 -> Data Type Conversion6/1  "<SW_Regen_Disable>"
  RegenFaultVal/1 -> Data Type Conversion8/1
  Data Type Conversion4/1 -> Switch/3
  Supervisory  Control  Logic1/11(Chg) -> Terminator10/1
  Bus Selector4/1 -> Data Type Conversion7/1  "<SW_CS_ON>"
  Bus Selector4/2 -> Data Type Conversion5/1  "<SW_Engine_ON>"
  eSystemStatusValidity/1(Out1) -> Terminator1/1
  iceSystemStatusValidity/1(Out1) -> Terminator2/1
  Bus Selector/10 -> Supervisory  Control  Logic1/11(plugged)  "<NLG5_S_CP_DT>"
  Bus Selector3/1 -> Supervisory  Control  Logic1/18(DrvIntdAxleTrq)  "<DrvIntndAxlTrq>"
  Bus Selector3/2 -> Supervisory  Control  Logic1/19(IntdAxleTrq)  "<FullDrvIntndAxlTrq>"
  ABSAtvVal/1 -> Data Type Conversion1/1
  Data Type Conversion1/1 -> Supervisory  Control  Logic1/27(ABSAtv)
  Subsystem1/1(Faked_SoC) -> Supervisory  Control  Logic1/20(Faked_SoC)
  Key_Position/1 -> Data Type Conversion2/1
  Data Type Conversion2/1 -> Switch/1
  Key_PosOvrd/1 -> Switch/2
  Switch/1 -> Supervisory  Control  Logic1/3(KeyPos)
  Supervisory  Control  Logic1/12(Brkmode) -> Bus Creator/17  "BrkMode"
  Supervisory  Control  Logic1/13(Drvmode) -> Bus Creator/18  "DrvMode"
  Data Type Conversion5/1 -> Switch3/3  "SWEnginePhys"
  Data Type Conversion6/1 -> Supervisory  Control  Logic1/24(RegenBrkDisable)
  Data Type Conversion7/1 -> Terminator3/1, Subsystem1/2(CS_On)  "SWCSPhys"
  Data Type Conversion8/1 -> Supervisory  Control  Logic1/28(Regen_fault)
  [BPP] -> Bus Creator/19
  Sports Mode Logic/1(Driver_Mode) -> Compare To Constant/1
  Bus Selector6/1 -> Supervisory  Control  Logic1/29(EngFdbkTrq)  "<EngActStdyStTorq>"
  Subsystem/1(Out1) -> Bus Creator/9  "MtrTrqCmdOut"
  Compare To Constant1/1 -> Bus Creator/1  "SportsModeEnable"
  [MotorSpeed] -> rad/s to RPM/1
  iceSystemStatusVal/1 -> Supervisory  Control  Logic1/26(iceSystemStatus)
  eSystemStatusVal/1 -> Supervisory  Control  Logic1/25(eSystemStatus)
  [BMS_Fehler_Pilot] -> SysPwrMd/4(Fehler_Pilot)
  Bus Selector6/2 -> Supervisory  Control  Logic1/30(EngCtlTmp)  "<EngCltTmp>"
  Data Type Conversion/1 -> Bus Creator/4  "closeMaincReq"
  Data Type Conversion9/1 -> Bus Creator/12  "HV_req"
  Data Type Conversion12/1 -> [Cdmode], Supervisory  Control  Logic1/31(CDmode)
  Bus Selector7/1 -> Supervisory  Control  Logic1/32(INV_State)  "<INV_State>"
  [Cdmode] -> Bus Creator/20  "CDmodeSW"
  Supervisory  Control  Logic1/7(MotTrqReq) -> IdealMotTrq/1(TrqCmd)  "MtrTrqCmd"
  IdealMotTrq/1(Out1) -> AxlTrq_to_MotTrq/1(In1)
  Memory/1 -> Data Type Conversion/1
  Memory1/1 -> Data Type Conversion9/1
  Bus Selector1/3 -> Supervisory  Control  Logic1/17(Voltage)  "<BMS_IstSpannung>"
  [AccPos_Perc] -> IdealMotTrq/2(APP)
  [Cdmode] -> IdealMotTrq/3(CDmode)
  [MotorSpeed] -> IdealMotTrq/4(FeedbackSpd)
  Bus Selector5/1 -> Sports Mode Logic/1(Voltage_Input)  "<Sport_Mode_SW>"
  Sensors/1 -> Bus Selector5/1, Bus Selector/1, Bus Selector10/1, Bus Selector7/1, Bus Selector8/1, Bus Selector9/1, Bus Selector6/1, Bus Selector4/1, Bus Selector1/1
  Bus Selector8/1 -> Data Type Conversion13/1  "<SW_Engine_ON>"
  EngineCharge Logic/1(CDmodeSW) -> Switch2/3  "CDmodeSWSF"
  Data Type Conversion13/1 -> ?
  Switch2/1 -> Data Type Conversion12/1
  CDmodeSW/1 -> Switch2/1
  CDmodeSWOvrrd/1 -> Switch2/2
  Bus Selector9/1 -> [BMS_Fehler_Pilot]  "<BMS_Fehler_Pilot>"
  Switch3/1 -> Supervisory  Control  Logic1/23(SW_Engine_ON)
  EngineONSW/1 -> Switch3/1
  EngineONOvrrd/1 -> Switch3/2
  Hood_Status/1(HoodStatus) -> Terminator/1
  [BPP] -> IdealMotTrq/5(BPP)
  Data Type Conversion11/1 -> ?
  Bus Selector8/2 -> Data Type Conversion11/1  "<SW_CS_ON>"
  AxlTrq_to_MotTrq/1(Out1) -> Subsystem/1(In1)
  [TransShftLvrPos] -> IdealMotTrq/6(ShifterPosition)
  Bus Selector10/1 -> Supervisory  Control  Logic1/34(IstModus)  "<BMS_IstModus>"
  Constant/1 -> Supervisory  Control  Logic1/33(HoodStatus)
  CDmodeSW1/1 -> EngineCharge Logic/1(SW_Engine_On)
  CDmodeSW2/1 -> EngineCharge Logic/2(SW_CS_On)
  SW_CS_ON/1 -> Data Type Conversion10/1
  Supervisory  Control  Logic1/5(EngAppReq) -> Bus Creator/7  "EngAppReq"
  Data Type Conversion10/1 -> Supervisory  Control  Logic1/22(SW_CS_ON)
  rad/s to RPM/1 -> Subsystem/2(RPM)

== system Hybrid_P2_Parallel_ETE/Sensors/CAN/EBCAN/BMS_Antrieb ==
  In1 : Inport
  Bus Creator : BusCreator  Inputs=2
  Bus Selector : BusSelector  OutputSignals=NMH_BMS,ISO_Hybrid_01_Resp
  ISO_Hybrid_01_Resp : Subsystem
  NMH_BMS : Subsystem
  Out1 : Outport
  wires:
  Bus Selector/2 -> ISO_Hybrid_01_Resp/1(In1)  "<ISO_Hybrid_01_Resp>"
  Bus Creator/1 -> Out1/1
  ISO_Hybrid_01_Resp/1(Out1) -> Bus Creator/2
  NMH_BMS/1(Out1) -> Bus Creator/1
  Bus Selector/1 -> NMH_BMS/1(In1)  "<NMH_BMS>"
  In1/1 -> Bus Selector/1

== system Hybrid_P2_Parallel_ETE/Sensors/CAN/EBCAN/CCM ==
  In1 : Inport
  Bus Creator : BusCreator  Inputs=2
  Bus Selector : BusSelector  OutputSignals=NMH_BMS,ISO_Hybrid_01_Resp
  ISO_Hybrid_01_Resp : Subsystem
  NMH_BMS : Subsystem
  Out1 : Outport
  wires:
  In1/1 -> Bus Selector/1
  Bus Selector/1 -> NMH_BMS/1(In1)  "<NMH_BMS>"
  NMH_BMS/1(Out1) -> Bus Creator/1
  ISO_Hybrid_01_Resp/1(Out1) -> Bus Creator/2
  Bus Creator/1 -> Out1/1
  Bus Selector/2 -> ISO_Hybrid_01_Resp/1(In1)  "<ISO_Hybrid_01_Resp>"

== system Hybrid_P2_Parallel_ETE/Sensors/CAN/EBCAN/ECM ==
  In1 : Inport
  Bus Creator : BusCreator  Inputs=7
  Bus Selector : BusSelector  OutputSignals=Sensors_to_ECM.EngActStdyStTorq_Nm,Sensors_to_ECM.EngSpd_RPM,ECM_to_Actuators.VehSpdAvgDrvn,ECM_to_Actuators.EngRunAtv,ECM_to_Actuators.Eng_Temp,ECM_to_Actuators.ECM_RollingAliveCnt
  Data Type Conversion{1..6} (6 alike) : DataTypeConversion
  ETEI_Engine_Torque_Status : Subsystem
  Ground : Ground
  PPEI_Engine_General_Status_4 : Subsystem
  PPEI_Engine_General_Status_6 : Subsystem
  PPEI_Vehicle_Speed_and_Distance : Subsystem
  PTEI_Engine_Torque_Status : Subsystem
  Out1 : Outport
  wires:
  Data Type Conversion1/1 -> Bus Creator/4  "EngRunAtv"
  Data Type Conversion3/1 -> Bus Creator/2  "EngSpd"
  PPEI_Engine_General_Status_6/1(Out1) -> Bus Creator/7
  Data Type Conversion6/1 -> PPEI_Engine_General_Status_6/1(In1)
  PPEI_Engine_General_Status_4/1(Out1) -> Bus Creator/6
  Data Type Conversion5/1 -> PPEI_Engine_General_Status_4/1(In1)
  PTEI_Engine_Torque_Status/1(Out1) -> Bus Creator/5
  Ground/1 -> PTEI_Engine_Torque_Status/1(In1)
  Bus Selector/4 -> Data Type Conversion1/1  "<EngRunAtv>"
  Bus Creator/1 -> Out1/1
  PPEI_Vehicle_Speed_and_Distance/1(Out1) -> Bus Creator/3
  ETEI_Engine_Torque_Status/1(Out1) -> Bus Creator/1
  Data Type Conversion4/1 -> PPEI_Vehicle_Speed_and_Distance/1(In1)
  Bus Selector/2 -> Data Type Conversion3/1  "<EngSpd_RPM>"
  Data Type Conversion2/1 -> ETEI_Engine_Torque_Status/1(In1)
  In1/1 -> Bus Selector/1
  Bus Selector/1 -> Data Type Conversion2/1  "<EngActStdyStTorq_Nm>"
  Bus Selector/3 -> Data Type Conversion4/1  "<VehSpdAvgDrvn>"
  Bus Selector/5 -> Data Type Conversion5/1  "<Eng_Temp>"
  Bus Selector/6 -> Data Type Conversion6/1  "<ECM_RollingAliveCnt>"

== system Hybrid_P2_Parallel_ETE/Sensors/CAN/HV_CAN/BMS_Hybrid ==
  In1 : Inport
  BMS_HYB_02 : Subsystem
  BMS_HYB_03 : Subsystem
  BMS_HYB_04 : Subsystem
  Bus Creator : BusCreator  Inputs=6
  Bus Selector : BusSelector  OutputSignals=BMS_HYB_02,BMS_HYB_04,BMS_HYB_03,BMS_HYB_02.BMS_Fehler_Isolation,BMS_HYB_06.BMS_Temperatur,BMS_HYB_02.BMS_Fehler_HS_verschweisst
  Data Type Conversion : DataTypeConversion
  Data Type Conversion1 : DataTypeConversion
  Data Type Conversion2 : DataTypeConversion
  Out1 : Outport
  wires:
  Data Type Conversion2/1 -> Bus Creator/6  "BMS_Fehler_HS_verschweisst"
  Bus Selector/5 -> Data Type Conversion/1  "<BMS_Temperatur>"
  Bus Selector/4 -> Data Type Conversion1/1  "<BMS_Fehler_Isolation>"
  BMS_HYB_03/1(Out1) -> Bus Creator/3
  Bus Selector/3 -> BMS_HYB_03/1(In1)  "<BMS_HYB_03>"
  BMS_HYB_04/1(Out1) -> Bus Creator/2
  BMS_HYB_02/1(Out1) -> Bus Creator/1
  Bus Creator/1 -> Out1/1
  Bus Selector/2 -> BMS_HYB_04/1(In1)  "<BMS_HYB_04>"
  Bus Selector/1 -> BMS_HYB_02/1(In1)  "<BMS_HYB_02>"
  In1/1 -> Bus Selector/1
  Data Type Conversion/1 -> Bus Creator/5  "BMS_Temperatur"
  Data Type Conversion1/1 -> Bus Creator/4  "BMS_Fehler_Isolation"
  Bus Selector/6 -> Data Type Conversion2/1  "<BMS_Fehler_HS_verschweisst>"

== system Hybrid_P2_Parallel_ETE/Sensors/CAN/HV_CAN/MCU ==
  In1 : Inport
  Bus Creator : BusCreator  Inputs=6
  Bus Creator1 : BusCreator  Inputs=2
  Bus Creator2 : BusCreator  Inputs=2
  Bus Selector : BusSelector  OutputSignals=Sensors_to_MCU.mot_spd_out,Sensors_to_MCU.mot_crr_out,MCU_to _Actuator.InverterEnabled,MCU_to _Actuator.MotTrqFdbck,MCU_to _Actuator.D3_Power_On_Timer,Sensors_to_MCU.mot_volt_in
  Bus Selector1 : BusSelector  OutputSignals=Sensors_to_MCU.mcu_temp,Sensors_to_MCU.mot_temp
  Data Type Conversion{1..5,7..9} (8 alike) : DataTypeConversion
  In2 : InportShadow
  Out1 : Outport
  wires:
  In1/1 -> Bus Selector/1
  Bus Selector/6 -> Data Type Conversion9/1  "<mot_volt_in>"
  Bus Selector/4 -> Data Type Conversion7/1  "<MotTrqFdbck>"
  Bus Selector/5 -> Data Type Conversion8/1  "<D3_Power_On_Timer>"
  Bus Creator/1 -> Bus Creator1/1  "INV_VCU_01"
  Data Type Conversion3/1 -> Bus Creator/3  "INV_State"
  Data Type Conversion2/1 -> Bus Creator/2  "INV_CurrentHV"
  Data Type Conversion1/1 -> Bus Creator/1  "INV_Speed"
  Bus Selector/3 -> Data Type Conversion3/1  "<InverterEnabled>"
  Bus Selector/2 -> Data Type Conversion2/1  "<mot_crr_out>"
  Bus Selector/1 -> Data Type Conversion1/1  "<mot_spd_out>"
  Data Type Conversion7/1 -> Bus Creator/4  "INV_OutputTorque"
  Data Type Conversion8/1 -> Bus Creator/5  "MessageCounter_200"
  Data Type Conversion9/1 -> Bus Creator/6  "INV_VoltageHV"
  Data Type Conversion4/1 -> Bus Creator2/1  "INV_InverterTemperature"
  Bus Selector1/2 -> Data Type Conversion5/1  "<mot_temp>"
  Data Type Conversion5/1 -> Bus Creator2/2  "INV_ElectricMachineTemperature"
  Bus Selector1/1 -> Data Type Conversion4/1  "<mcu_temp>"
  In2/1 -> Bus Selector1/1
  Bus Creator2/1 -> Bus Creator1/2  "INV_VCU_04"
  Bus Creator1/1 -> Out1/1

== system Hybrid_P2_Parallel_ETE/Sensors/CAN/HV_CAN/OBC ==
  In1 : Inport
  Bus Creator : BusCreator  Inputs=5
  Bus Selector : BusSelector  OutputSignals=NLG5_ACT_I,NLG5_ACT_II,NLG5_ERR,NLG5_ST,NLG5_TEMP
  NLG5_ACT_I : Subsystem
  NLG5_ACT_II : Subsystem
  NLG5_ERR : Subsystem
  NLG5_ST : Subsystem
  NLG5_TEMP : Subsystem
  Out1 : Outport
  wires:
  In1/1 -> Bus Selector/1
  Bus Selector/1 -> NLG5_ACT_I/1(In1)  "<NLG5_ACT_I>"
  NLG5_ACT_I/1(Out1) -> Bus Creator/1
  Bus Selector/2 -> NLG5_ACT_II/1(In1)  "<NLG5_ACT_II>"
  NLG5_ACT_II/1(Out1) -> Bus Creator/2
  NLG5_ERR/1(Out1) -> Bus Creator/3
  Bus Selector/3 -> NLG5_ERR/1(In1)  "<NLG5_ERR>"
  Bus Selector/4 -> NLG5_ST/1(In1)  "<NLG5_ST>"
  NLG5_ST/1(Out1) -> Bus Creator/4
  Bus Selector/5 -> NLG5_TEMP/1(In1)  "<NLG5_TEMP>"
  NLG5_TEMP/1(Out1) -> Bus Creator/5
  Bus Creator/1 -> Out1/1

== system Hybrid_P2_Parallel_ETE/Sensors/CAN/VEH_CAN/BCM ==
  In1 : Inport
  Bus Creator : BusCreator  Inputs=2
  Bus Selector : BusSelector  OutputSignals=SysPwrMd,BrkPdlPos
  Data Type Conversion : DataTypeConversion
  Data Type Conversion1 : DataTypeConversion
  PPEI_Brake_Apply_Status : Subsystem
  PPEI_Platfrom_General_Status : Subsystem
  Out1 : Outport
  wires:
  Data Type Conversion1/1 -> PPEI_Brake_Apply_Status/1(In1)
  Data Type Conversion/1 -> PPEI_Platfrom_General_Status/1(In1)
  Bus Creator/1 -> Out1/1
  PPEI_Brake_Apply_Status/1(Out1) -> Bus Creator/2
  PPEI_Platfrom_General_Status/1(Out1) -> Bus Creator/1
  Bus Selector/2 -> Data Type Conversion1/1  "<BrkPdlPos>"
  Bus Selector/1 -> Data Type Conversion/1  "<SysPwrMd>"
  In1/1 -> Bus Selector/1

== system Hybrid_P2_Parallel_ETE/Sensors/CAN/VEH_CAN/EBCM ==
  In1 : Inport
  Bus Selector : BusSelector  OutputSignals=PPEI_Chassis_General_Status_1.BrkPdlDrvAppPrsDetcd
  Constant : Constant  OutDataTypeStr=boolean
  PPEI_Chassis_General_Status_1 : Subsystem
  Terminator : Terminator
  Out1 : Outport
  wires:
  Constant/1 -> PPEI_Chassis_General_Status_1/1(In1)
  In1/1 -> Bus Selector/1
  PPEI_Chassis_General_Status_1/1(Out1) -> Out1/1
  Bus Selector/1 -> Terminator/1  "<BrkPdlDrvAppPrsDetcd>"

== system Hybrid_P2_Parallel_ETE/Sensors/CAN/VEH_CAN/ICCM ==
  In1 : Inport
  Out1 : Outport
  wires:
  In1/1 -> Out1/1

== system Hybrid_P2_Parallel_ETE/Sensors/CAN/VEH_CAN/TCM ==
  In1 : Inport
  Bus Creator : BusCreator  Inputs=4
  Bus Selector : BusSelector  OutputSignals=TCM_to _Actuator.TransEstGear,TCM_to _Actuator.LockupCmd,TCM_to _Actuator.TrnsShftLvrPos,Sensors_to_TCM.gb_trq_ratio
  Data Type Conversion{,1..3} (4 alike) : DataTypeConversion
  Out1 : Outport
  wires:
  Data Type Conversion/1 -> Bus Creator/1  "TransEstGear"
  Bus Creator/1 -> Out1/1
  In1/1 -> Bus Selector/1
  Data Type Conversion1/1 -> Bus Creator/2  "TrnsTrqCnvCltCmndMd"
  Data Type Conversion2/1 -> Bus Creator/3  "TrnsShftLvrPos"
  Data Type Conversion3/1 -> Bus Creator/4  "TrnGrRat"
  Bus Selector/1 -> Data Type Conversion/1  "<TransEstGear>"
  Bus Selector/2 -> Data Type Conversion1/1  "<LockupCmd>"
  Bus Selector/3 -> Data Type Conversion2/1  "<TrnsShftLvrPos>"
  Bus Selector/4 -> Data Type Conversion3/1  "<gb_trq_ratio>"

== system Hybrid_P2_Parallel_ETE/Camaro Plant Model/E-Machine/IMG Plant/Electric Machine/Calculate Mot Efficiency, MotPwrMech, and, MotPwrElec1 ==
  note: Pelec_req = Pmech_req*Eff^k,
      | k = -1 if Trq >= 0,
      | k = 1 if Trq < 0
  MotSpd : Inport
  MotTrqAct : Inport  Port=2
  -1 : Gain  Gain=8
  "-1 when + 1 when - " : Gain  Gain=-1
  -2 : Gain  Gain=tloop
  2-D Lookup Table : Lookup_n-D  BreakpointsForDimension1=mot.plant.init.eff_trq.idx2_trq  BreakpointsForDimension2=mot.plant.init.eff_trq.idx1_spd  Table=mot.plant.init.eff_trq.map  InternalRulePriority=Speed  RndMeth=Simplest  InputSameDT=on
  Abs{,1..3} (4 alike) : Abs
  Add : Sum  Inputs=-+
  Add1 : Sum  Inputs=+-
  Constant : Constant  Value=1-0.8
  Gain2 : Gain  Gain=1/100
  MCU_WEGPmp : Constant  Value=0
  Math Function1 : Math  Operator=pow  SaturateOnIntegerOverflow=on
  Memory : Memory
  Product : Product
  Product1 : Product
  Product2 : Product
  Sign : Signum
  rad/s to rpm : Gain  Gain=30/pi
  Losses : Outport
  MCU_Heat : Outport  Port=2
  MotPwrElec : Outport  Port=3
  wires:
  -2/1 -> MCU_Heat/1
  -1/1 -> Add1/2
  Add1/1 -> -2/1
  MCU_WEGPmp/1 -> -1/1
  Abs3/1 -> Add1/1
  Product2/1 -> Abs3/1
  Constant/1 -> Product2/2
  Memory/1 -> Sign/1
  Math Function1/1 -> Product1/2
  Add/1 -> Abs2/1
  Abs2/1 -> Losses/1
  "-1 when + 1 when - "/1 -> Math Function1/2
  MotSpd/1 -> rad/s to rpm/1, Product/2
  MotTrqAct/1 -> Abs/1, Product/1, Memory/1
  Product/1 -> Product1/1, Add/1  "MotPwrMech"
  Product1/1 -> Add/2, Product2/1, MotPwrElec/1  "MotPwrElec"
  2-D Lookup Table/1 -> Gain2/1
  Gain2/1 -> Math Function1/1
  Abs/1 -> 2-D Lookup Table/1
  Sign/1 -> "-1 when + 1 when - "/1
  Abs1/1 -> 2-D Lookup Table/2
  rad/s to rpm/1 -> Abs1/1
